simulink model "ABS_Pole_Placement_Control"  (R2024b)
settings: Solver=VariableStepAuto  StartTime=0.0  StopTime=3  RelTol=1e-3
values from neighbouring files (symbols this model uses):
  Ad_pem = M_n4sid_pem.A    [ABS_Pole_Placement.m]
  Bd_pem = M_n4sid_pem.B    [ABS_Pole_Placement.m]
  Cd_pem = M_n4sid_pem.C    [ABS_Pole_Placement.m]
  Dd_pem = M_n4sid_pem.D    [ABS_Pole_Placement.m]
  K = dlqr(Ad, Bd, Q, R)    [ABS_LQR.m]    (also in ABS_Pole_Placement.m = place(Ad_pem, Bd_pem, poli_doriti))
settings Model: Creator=Octavian  LastModifiedBy=Octavian

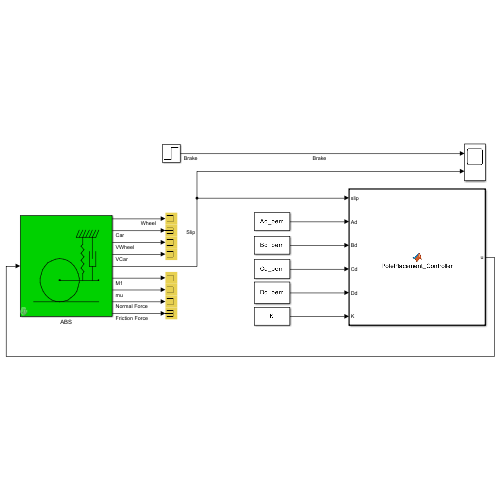
[thumbnail: Simulink's stored preview of the top-level diagram]
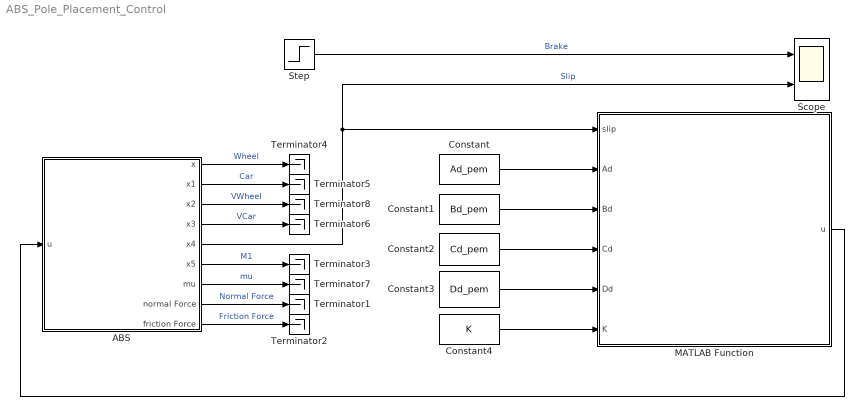
== system ABS_Pole_Placement_Control ==
  ABS : Subsystem  mask{r=[99.5 99]*1e-3, J=[7.5281 25.603]*1e-3, d=[1.2 2.25]*1e-4, M=[3  93]*1e-3, Mg=19.6181, w=[-0.04240011450454   0.00000000029375   0.03508217905067   0.40662691102315], p=2.09945271667129, a=0.00025724985785, L=0.370, phi=65.61*pi/180, uu=[0.40748031496063 15.24 -6.21], tau=0.048, xini=[180 180 0]}
      mask prompts: r "r1, r2"; J "J1, J2"; d "d1, d2"; M "M10, M20"; uu "brake param. u0, b1 b2"; tau "tau (c31=1/tau)"; xini "xini = [x1(0) x2(0) x3(0)]"
      mask init:
      | J1 = J(1);J2 = J(2);d1 = d(1);d2=d(2);r1 = r(1);r2=r(2);M10 = M(1);M20 = M(2);u0 = uu(1);b1 = uu(2);b2=uu(3);
      mask Display: plot([-0.2 -0.2], [-0.2 -0.2], [1.2 1.2], [1.2 1.2], [0.9 0.9], [0.6 0.9], [0.9 0.9], [0.3 0.5], [0.85 0.85 0.95 0.95], [0.7 0.5 0.5 0.7], [0.75 0.75], [0.8 0.9], [0.75 0.75], [0.3 0.4], [0.75 0.775], [0.4 0.425], [0.775 0.725 0.775], [0.425 0.475 0.525], [0.775 0.725 0.775], [0.525 0.575 0.625], [0.775 0.725 0.775], [0.625 0.675 0.725], [0.775 0.725 0.75], [0.725 0.775 0.8], [0.65 0.95], [0.9 0.9], [0.65 0.7], [0.9 1], [0.7 0.75], [0.9 1], [0.75 0.8], [0.9 1], [0.8 0.85], [0.9 1], [0.85 0.9], [0.9 1], [0.9 0.95], [0.9 1], [0.95 1], [0.9 1], 0.4+0.3*sin([0 0.20 0.41 0.62 0.83 1.04 1.25 1.46 1.67 1.88 2.09 2.30 2.51 2.72 2.93 3.14 3.35 3.56 3.76 3.97 4.18 4.39 4.60 4.81 5.02 5.23 5.44 5.65 5.86 6.07 6.28]), 0.3+0.3*cos([0 0.20 0.41 0.62 0.83 1.04 1.25 1.46 1.67 1.88 2.09 2.30 2.51 2.72 2.93 3.14 3.35 3.56 3.76 3.97 4.18 4.39 4.60 4.81 5.02 5.23 5.44 5.65 5.86 6.07 6.28]), (1-0.005)+0.005*sin([0 0.20 0.41 0.62 0.83 1.04 1.25 1.46 1.67 1.88 2.09 2.30 2.51 2.72 2.93 3.14 3.35 3.56 3.76 3.97 4.18 4.39 4.60 4.81 5.02 5.23 5.44 5.65 5.86 6.07 6.28]), 0.3+0.005*cos([0 0.20 0.41 0.62 0.83 1.04 1.25 1.46 1.67 1.88 2.09 2.30 2.51 2.72 2.93 3.14 3.35 3.56 3.76 3.97 4.18 4.39 4.60 4.81 5.02 5.23 5.44 5.65 5.86 6.07 6.28]), 0.4+0.005*sin([0 0.20 0.41 0.62 0.83 1.04 1.25 1.46 1.67 1.88 2.09 2.30 2.51 2.72 2.93 3.14 3.35 3.56 3.76 3.97 4.18 4.39 4.60 4.81 5.02 5.23 5.44 5.65 5.86 6.07 6.28]), 0.3+0.005*cos([0 0.20 0.41 0.62 0.83 1.04 1.25 1.46 1.67 1.88 2.09 2.30 2.51 2.72 2.93 3.14 3.35 3.56 3.76 3.97 4.18 4.39 4.60 4.81 5.02 5.23 5.44 5.65 5.86 6.07 6.28]), [0.4 1], [0.3 0.3], [0 1], [0 0] )
  Constant : Constant  Value=Ad_pem  OutDataTypeStr=double  SampleTime=0.0091
  Constant1 : Constant  Value=Bd_pem  OutDataTypeStr=double  SampleTime=0.0091
  Constant2 : Constant  Value=Cd_pem  OutDataTypeStr=double  SampleTime=0.0091
  Constant3 : Constant  Value=Dd_pem  SampleTime=0.0091
  Constant4 : Constant  Value=K  OutDataTypeStr=double  SampleTime=0.0091
  MATLAB Function : MATLAB Function  TreatAsAtomicUnit=on
  Scope : Scope  NumInputPorts=2
  Step : Step  Time=0  SampleTime=0.0091
  Terminator{1..8} (8 alike) : Terminator
  wires:
  ABS/7(mu) -> Terminator7/1  "mu"
  ABS/2(x1) -> Terminator5/1  "Car"
  Step/1 -> Scope/1  "Brake"
  ABS/9(friction Force) -> Terminator2/1  "Friction Force"
  ABS/3(x2) -> Terminator8/1  "VWheel"
  ABS/8(normal Force) -> Terminator1/1  "Normal Force"
  ABS/1(x) -> Terminator4/1  "Wheel"
  ABS/5(x4) -> MATLAB Function/1(slip), Scope/2  "Slip"
  ABS/4(x3) -> Terminator6/1  "VCar"
  ABS/6(x5) -> Terminator3/1  "M1"
  MATLAB Function/1(u) -> ABS/1(u)
  Constant/1 -> MATLAB Function/2(Ad)
  Constant1/1 -> MATLAB Function/3(Bd)
  Constant2/1 -> MATLAB Function/4(Cd)
  Constant3/1 -> MATLAB Function/5(Dd)
  Constant4/1 -> MATLAB Function/6(K)

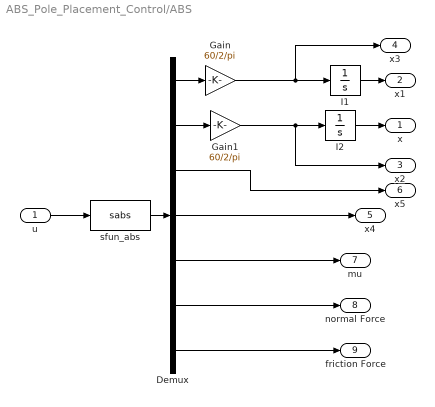
== system ABS_Pole_Placement_Control/ABS ==
  u : Inport
  Demux : Demux  Outputs=7
      settings: DisplayOption=none
  Gain : Gain  Gain=60/2/pi  SaturateOnIntegerOverflow=on  OutDataTypeStr=Inherit: Same as input  ParamDataTypeStr=Inherit: Same as input
  Gain1 : Gain  Gain=60/2/pi  SaturateOnIntegerOverflow=on  OutDataTypeStr=Inherit: Same as input  ParamDataTypeStr=Inherit: Same as input
  I1 : Integrator
  I2 : Integrator
  sfun_abs : S-Function  FunctionName=sabs  Parameters=r1,r2,J1,J2,d1,d2,M10,M20,Mg,w,p,a,L,phi,u0,b1,b2,tau,xini  SFunctionDeploymentMode=off  EnableBusSupport=off
  x : Outport
  x1 : Outport  Port=2
  x2 : Outport  Port=3
  x3 : Outport  Port=4
  x4 : Outport  Port=5
  x5 : Outport  Port=6
  mu : Outport  Port=7
  normal Force : Outport  Port=8
  friction Force : Outport  Port=9
  wires:
  u/1 -> sfun_abs/1
  sfun_abs/1 -> Demux/1
  Demux/1 -> Gain/1
  Gain/1 -> I1/1, x3/1
  Demux/2 -> Gain1/1
  Gain1/1 -> I2/1, x2/1
  I1/1 -> x1/1
  I2/1 -> x/1
  Demux/4 -> x4/1
  Demux/3 -> x5/1
  Demux/5 -> mu/1
  Demux/6 -> normal Force/1
  Demux/7 -> friction Force/1

== matlab function ABS_Pole_Placement_Control/MATLAB Function ==
  settings: updateMethod=DISCRETE  sampleTime=0.0091
  data: slip input double size=[1 1]; Ad input double size=[2 2]; Bd input double size=[2 1]; Cd input double size=[1 2]; Dd input double size=[1 1]; K input size=[1 2]; u output double size=[1 1]
function u = PolePlacement_Controller(slip, Ad, Bd, Cd, Dd, K)

persistent x

if isempty(x)
    x = zeros(size(Ad,1), 1);  
end

slip_ref = 0.82;  % Referință ideală

% Eroare de urmărire
e = slip_ref - slip;

% Câștig proporțional pe eroare
Ke = 0.8;  % <-- ajustează-l între 0.5 și 1.0 după nevoie

u_k = -K * x + Ke * e;

u = max(0, min(1, u_k));
x = Ad * x + Bd * u;
end
